simulink model "Testkinematic"  (R2019a)
settings: Solver=ode45  StartTime=0.0  StopTime=9  RelTol=1e-3  EnableMultiTasking=on
values from neighbouring files (symbols this model uses):
  x0 = 0    [Testkinematiccontrol.m]
settings Model: Creator=Gu  LastModifiedBy=ADMIN
settings DataIOCC: LimitDataPoints=on  SaveFormat=Array  ReturnWorkspaceOutputs=off
settings OptimizationCC: ExpressionDepthLimit=2147483647  LifeSpan=inf
settings DebuggingCC: UnderspecifiedInitializationDetection=Classic  MergeDetectMultiDrivingBlocksExec=none  FcnCallInpInsideContextMsg=warning  StateNameClashWarn=warning  SFUnexpectedBacktrackingDiag=warning  SFNoUnconditionalDefaultTransitionDiag=warning  SFExecutionAtInitializationDiag=none  ArithmeticOperatorsInVariantConditions=warning
settings HardwareCC: ProdBitPerPointer=32  ProdBitPerSizeT=32  ProdBitPerPtrDiffT=32  ProdLargestAtomicFloat=None  ProdIntDivRoundTo=Undefined  ProdEndianess=Unspecified  ProdWordSize=32  ProdHWDeviceType=32-bit Generic
settings ModelReferenceCC: PropagateSignalLabelsOutOfModel=off
settings SFSimCC: SimUseLocalCustomCode=off  SimParseCustomCode=off
settings RTWCC: RTWUseLocalCustomCode=off
settings CodeAppCC: StateflowObjectComments=on
settings GRTTargetCC: TargetLangStandard=C89/C90 (ANSI)  CombineOutputUpdateFcns=off  GRTInterface=on
settings ConfigComp: CovMetricSettings=dw  CovSaveCumulativeToWorkspaceVar=on  CovSaveSingleToWorkspaceVar=on  CovExternalEMLEnable=off  CovSFcnEnable=off

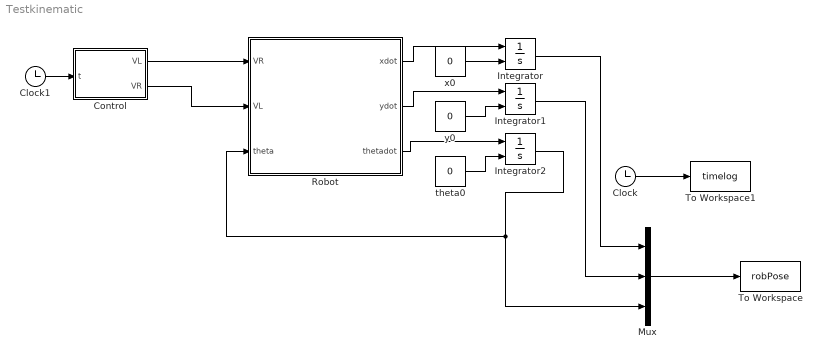
== system Testkinematic ==
  Clock : Clock
  Clock1 : Clock
  Control : MATLAB Function  TreatAsAtomicUnit=on
  Integrator : Integrator  InitialConditionSource=external  InitialCondition=x0
  Integrator1 : Integrator  InitialConditionSource=external  InitialCondition=2
  Integrator2 : Integrator  InitialConditionSource=external  InitialCondition=pi/4
  Mux : Mux  Inputs=3
  Robot : MATLAB Function  TreatAsAtomicUnit=on
  To Workspace : ToWorkspace  VariableName=robPose  SampleTime=0.1
  To Workspace1 : ToWorkspace  VariableName=timelog  SampleTime=-1
      settings: Save2DSignal=2-D array (concatenate along first dimension)
  theta0 : Constant  Value=0
  x0 : Constant  Value=0
  y0 : Constant  Value=0
  wires:
  Robot/1(xdot) -> Integrator/1
  Robot/2(ydot) -> Integrator1/1
  Robot/3(thetadot) -> Integrator2/1
  Integrator2/1 -> Robot/3(theta), Mux/3
  Integrator/1 -> Mux/1
  Integrator1/1 -> Mux/2
  Clock/1 -> To Workspace1/1
  Mux/1 -> To Workspace/1
  Control/1(VL) -> Robot/1(VR)
  Control/2(VR) -> Robot/2(VL)
  Clock1/1 -> Control/1(t)
  x0/1 -> Integrator/2
  y0/1 -> Integrator1/2
  theta0/1 -> Integrator2/2

== matlab function Testkinematic/Control ==
  data: t input; VL output; VR output
function [VL,VR]= fcn(t)
if t<=2
    VL=0.1;
    VR=0.1;
elseif t>2 && t<=5
    VL=0.1;
    VR=0.05;
else 
    VL=0.05;
    VR=0.1;
end

== matlab function Testkinematic/Robot ==
  data: VR input; xdot output; VL input; theta input; ydot output; thetadot output
function [xdot, ydot, thetadot] = fcn(VR, VL,theta)

d=0.08325*2; 
xdot=(VR+VL)/2*cos(theta);
ydot=(VR+VL)/2*sin(theta);
thetadot=(VR-VL)/d;
